simulink model "sfcndemo_counter_cpp"  (Simulink 6.0)
settings: Solver=FixedStepDiscrete  StartTime=0.0  StopTime=9.9  FixedStep=1  RelTol=1e-3
settings Model: Creator=The MathWorks Inc.  LastModifiedBy=batserve  ExtModeTrigMode=oneshot  ExtModeArmWhenConnect=off  ExtModeAutoUpdateStatusClock=off
settings DataIOCC: LimitDataPoints=off
settings OptimizationCC: BlockReduction=off  BooleanDataType=off
settings DebuggingCC: CheckExecutionContextPreStartOutputMsg=on  CheckExecutionContextRuntimeOutputMsg=on  SolverPrmCheckMsg=none
settings HardwareCC: TargetUnknown=on
settings RTWCC: SystemTargetFile=cpptarget.tlc  TemplateMakefile=cpp_unix.tmf  RetainRTWFile=on  ProcessScript=cpptarget_make_rtw_hook
settings STFCustomTargetCC: TargetFcnLib=ansi_tfl_tmw.mat  GenFloatMathFcnCalls=ANSI_C  ModelReferenceCompliant=off  CombineOutputUpdateFcns=on  MatFileLogging=on  SystemTargetFile=cpptarget.tlc

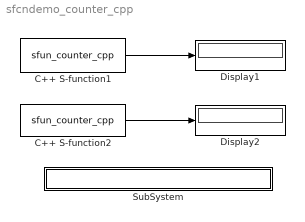
== system sfcndemo_counter_cpp ==
  C++ S-function1 : S-Function  FunctionName=sfun_counter_cpp  Parameters=1
  C++ S-function2 : S-Function  FunctionName=sfun_counter_cpp  Parameters=2
  Display1 : Display
  Display2 : Display
  SubSystem : Subsystem  PropExecContextAcrossSSBoundary=on
      settings: OpenFcn=edit(fullfile(matlabroot,'simulink','src','sfun_counter_cpp.cpp'));
      mask Display: disp('matlabroot\simulink\src\sfun_counter_cpp.cpp');
  wires:
  C++ S-function1/1 -> Display1/1
  C++ S-function2/1 -> Display2/1

== system sfcndemo_counter_cpp/SubSystem ==
